simulink model "task1"  (R2024a)
settings: Solver=VariableStepAuto  StartTime=0.0  StopTime=10  RelTol=1e-3
undefined symbols (not defined in the file): K_1, ss_plant_discrete, T
settings Model: Creator=vladislav  LastModifiedBy=lalayants

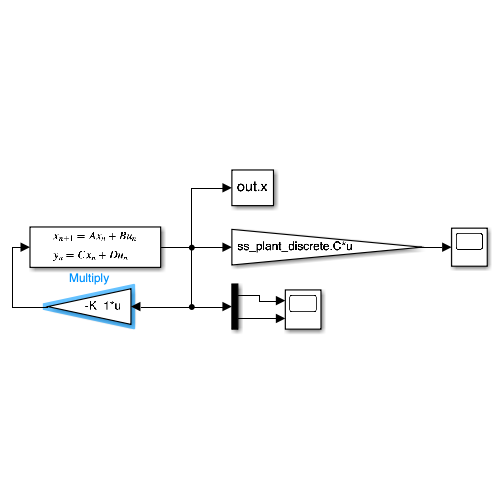
[thumbnail: Simulink's stored preview of the top-level diagram]
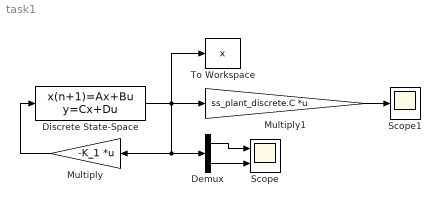
== system task1 ==
  Demux : Demux  Outputs=2
  Discrete State-Space : DiscreteStateSpace  A=ss_plant_discrete.A  B=ss_plant_discrete.B  C=eye(2)  D=[0; 0]  InitialCondition=[1 1]  SampleTime=T
  Multiply : Gain  Gain=-K_1  Multiplication=Matrix(K*u)
  Multiply1 : Gain  Gain=ss_plant_discrete.C  Multiplication=Matrix(K*u)
  Scope : Scope  NumInputPorts=2
  Scope1 : Scope
  To Workspace : ToWorkspace  VariableName=x  SaveFormat=Timeseries  SampleTime=-1
  wires:
  Discrete State-Space/1 -> To Workspace/1, Multiply1/1, Demux/1, Multiply/1
  Multiply/1 -> Discrete State-Space/1
  Demux/1 -> Scope/1
  Demux/2 -> Scope/2
  Multiply1/1 -> Scope1/1
